simulink model "loadModelAndPredict"  (Simulink 9.1)
settings: Solver=VariableStepAuto  StartTime=0.0  StopTime=1000  RelTol=1e-3
settings Model: Creator=18840  LastModifiedBy=18840
settings DataIOCC: SaveFormat=Dataset
settings OptimizationCC: LifeSpan=auto
settings DebuggingCC: UnderspecifiedInitializationDetection=Simplified  MergeDetectMultiDrivingBlocksExec=error  SFUnexpectedBacktrackingDiag=error  SFNoUnconditionalDefaultTransitionDiag=error  SFExecutionAtInitializationDiag=warning
settings HardwareCC: ProdBitPerPointer=64  ProdBitPerSizeT=64  ProdBitPerPtrDiffT=64  ProdLargestAtomicFloat=Float  ProdIntDivRoundTo=Zero  ProdEndianess=LittleEndian  ProdWordSize=64  ProdHWDeviceType=Intel->x86-64 (Windows64)
settings ModelReferenceCC: PropagateSignalLabelsOutOfModel=on
settings CodeAppCC: StateflowObjectComments=off
settings GRTTargetCC: TargetLangStandard=C99 (ISO)  CombineOutputUpdateFcns=on  GRTInterface=off
settings ConfigComp: CovMetricSettings=dwe  CovHtmlReporting=off  CovSaveCumulativeToWorkspaceVar=off  CovSaveSingleToWorkspaceVar=off  CovExternalEMLEnable=on

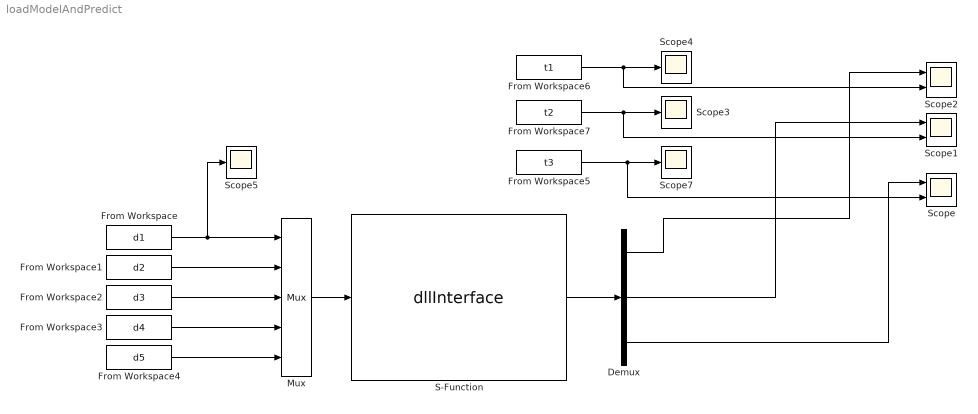
== system loadModelAndPredict ==
  Demux : Demux  Outputs=3
  From Workspace : FromWorkspace  VariableName=d1  SampleTime=0
  From Workspace1 : FromWorkspace  VariableName=d2  SampleTime=0
  From Workspace2 : FromWorkspace  VariableName=d3  SampleTime=0
  From Workspace3 : FromWorkspace  VariableName=d4  SampleTime=0
  From Workspace4 : FromWorkspace  VariableName=d5  SampleTime=0
  From Workspace5 : FromWorkspace  VariableName=t3  SampleTime=0
  From Workspace6 : FromWorkspace  VariableName=t1  SampleTime=0
  From Workspace7 : FromWorkspace  VariableName=t2  SampleTime=0
  Mux : Mux  Inputs=5
  S-Function : S-Function  FunctionName=dllInterface  Parameters=0.25  SFunctionDeploymentMode=off  EnableBusSupport=off
  Scope : Scope  NumInputPorts=2
  Scope1 : Scope  NumInputPorts=2
  Scope2 : Scope  NumInputPorts=2
  Scope{3..5,7} (4 alike) : Scope
  wires:
  Mux/1 -> S-Function/1
  Demux/2 -> Scope1/1
  Demux/3 -> Scope/1
  Demux/1 -> Scope2/1
  S-Function/1 -> Demux/1
  From Workspace1/1 -> Mux/2
  From Workspace2/1 -> Mux/3
  From Workspace/1 -> Scope5/1, Mux/1
  From Workspace4/1 -> Mux/5
  From Workspace3/1 -> Mux/4
  From Workspace5/1 -> Scope/2, Scope7/1
  From Workspace7/1 -> Scope1/2, Scope3/1
  From Workspace6/1 -> Scope2/2, Scope4/1
